simulink model "ROBOT_CONTROL_K2"  (R2023a)
settings: Solver=VariableStepAuto  StartTime=0.0  StopTime=10  RelTol=1e-3
values from neighbouring files (symbols this model uses):
  Bm = 0.015    [ROBOT_CONTROL.m]    (also in collaborative_class_main.m)
  g = 9.81    [ROBOT_CONTROL.m]    (also in collaborative_class_main.m)
  Jl = 4e-4    (= 0.0004)    [ROBOT_CONTROL.m]    (also in collaborative_class_main.m)
  Jm = 4e-4    (= 0.0004)    [ROBOT_CONTROL.m]    (also in collaborative_class_main.m)
  k = 0.8    [ROBOT_CONTROL.m]    (also in collaborative_class_main.m)
  l = 0.3    [ROBOT_CONTROL.m]    (also in collaborative_class_main.m)
  m = 0.3    [ROBOT_CONTROL.m]    (also in collaborative_class_main.m)
  u_bar = m*g*l*cos(x2_bar)    [ROBOT_CONTROL.m]
undefined symbols (not defined in the file or in its folder): const, Kv_tilde
settings Model: Creator=Kevin  LastModifiedBy=alexz

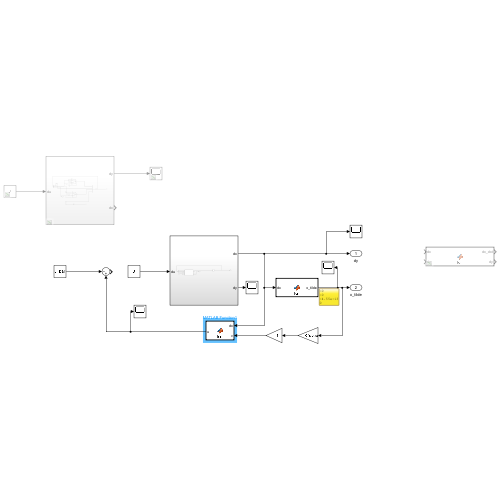
[thumbnail: Simulink's stored preview of the top-level diagram]
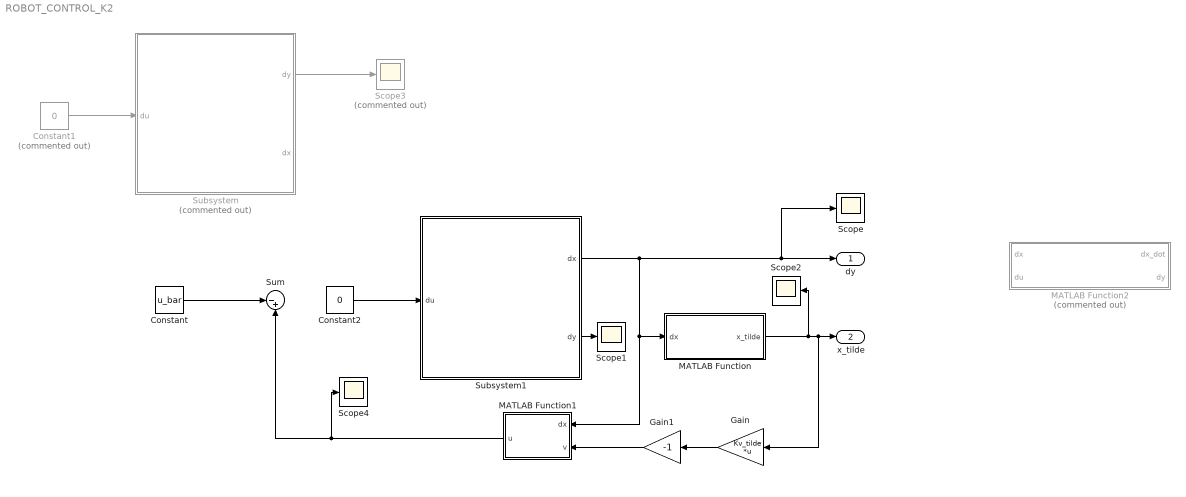
== system ROBOT_CONTROL_K2 ==
  Constant : Constant  Value=u_bar
  Constant1 : Constant  Commented=on  Value=0
  Constant2 : Constant  Value=0
  Gain : Gain  Gain=Kv_tilde  Multiplication=Matrix(K*u) (u vector)
  Gain1 : Gain  Gain=-1
  MATLAB Function : MATLAB Function  TreatAsAtomicUnit=on
  MATLAB Function1 : MATLAB Function  TreatAsAtomicUnit=on
  MATLAB Function2 : MATLAB Function  Commented=on  TreatAsAtomicUnit=on
  Scope{,1..2,4} (4 alike) : Scope
  Scope3 : Scope  Commented=on
  Subsystem : Subsystem  Commented=on
  Subsystem1 : Subsystem
  Sum : Sum  Inputs=|-+
  dy : Outport
  x_tilde : Outport  Port=2
  wires:
  Subsystem1/1(dx) -> MATLAB Function1/1(dx), MATLAB Function/1(dx), Scope/1, dy/1
  MATLAB Function/1(x_tilde) -> Scope2/1, Gain/1, x_tilde/1
  Gain/1 -> Gain1/1
  MATLAB Function1/1(u) -> Scope4/1, Sum/2
  Constant/1 -> Sum/1
  Gain1/1 -> MATLAB Function1/2(v)
  Subsystem1/2(dy) -> Scope1/1
  Constant1/1 -> Subsystem/1(du)
  Subsystem/1(dy) -> Scope3/1
  Constant2/1 -> Subsystem1/1(du)

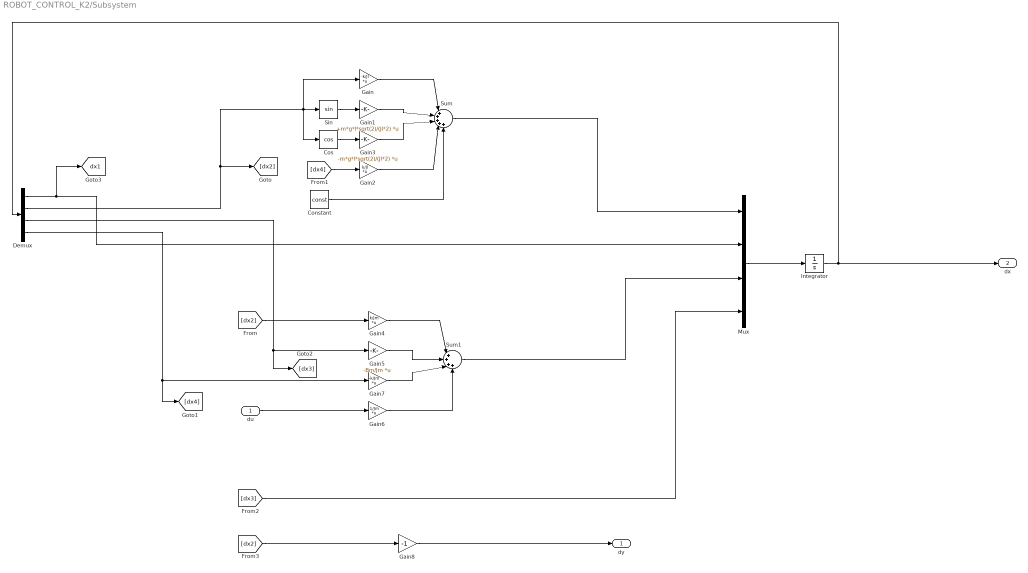
== system ROBOT_CONTROL_K2/Subsystem ==
  du : Inport
  Constant : Constant  Value=const
  Cos : Trigonometry  Operator=cos
  Demux : Demux
  Gain : Gain  Gain=-k/Jl  Multiplication=Matrix(K*u) (u vector)
  Gain1 : Gain  Gain=+m*g*l*sqrt(2)/(Jl*2)  Multiplication=Matrix(K*u) (u vector)
  Gain2 : Gain  Gain=k/Jl  Multiplication=Matrix(K*u) (u vector)
  Gain3 : Gain  Gain=-m*g*l*sqrt(2)/(Jl*2)  Multiplication=Matrix(K*u) (u vector)
  Gain4 : Gain  Gain=k/Jm  Multiplication=Matrix(K*u) (u vector)
  Gain5 : Gain  Gain=-Bm/Jm  Multiplication=Matrix(K*u) (u vector)
  Gain6 : Gain  Gain=1/Jm  Multiplication=Matrix(K*u) (u vector)
  Gain7 : Gain  Gain=-k/Jm  Multiplication=Matrix(K*u) (u vector)
  Gain8 : Gain  Gain=-1
  Integrator : Integrator
  Mux : Mux
  Sin : Trigonometry
  Sum : Sum  Inputs=|+++++
  Sum1 : Sum  Inputs=|++++
  dy : Outport
  dx : Outport  Port=2
  tag scope: dx1=global
  wires:
  [dx2] -> Gain4/1
  Gain6/1 -> Sum1/4
  Gain8/1 -> dy/1
  Demux/2 -> [dx2], Gain/1, Sin/1, Cos/1
  Gain1/1 -> Sum/2
  Constant/1 -> Sum/5
  Cos/1 -> Gain3/1
  Demux/3 -> [dx3], Gain5/1
  [dx4] -> Gain2/1
  Gain7/1 -> Sum1/3
  Sin/1 -> Gain1/1
  Demux/4 -> Gain7/1, [dx4]
  Gain3/1 -> Sum/3
  Sum1/1 -> Mux/3
  Gain4/1 -> Sum1/1
  Gain/1 -> Sum/1
  Gain5/1 -> Sum1/2
  Sum/1 -> Mux/1
  Gain2/1 -> Sum/4
  [dx3] -> Mux/4
  du/1 -> Gain6/1
  [dx2] -> Gain8/1
  Mux/1 -> Integrator/1
  Demux/1 -> [dx1], Mux/2
  Integrator/1 -> dx/1, Demux/1

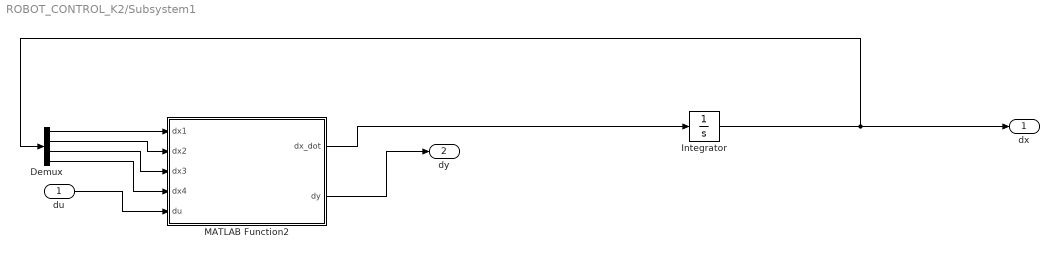
== system ROBOT_CONTROL_K2/Subsystem1 ==
  du : Inport
  Demux : Demux
  Integrator : Integrator
  MATLAB Function2 : MATLAB Function  TreatAsAtomicUnit=on
  dx : Outport
  dy : Outport  Port=2
  wires:
  Integrator/1 -> Demux/1, dx/1
  du/1 -> MATLAB Function2/5(du)
  MATLAB Function2/2(dy) -> dy/1
  MATLAB Function2/1(dx_dot) -> Integrator/1
  Demux/1 -> MATLAB Function2/1(dx1)
  Demux/2 -> MATLAB Function2/2(dx2)
  Demux/3 -> MATLAB Function2/3(dx3)
  Demux/4 -> MATLAB Function2/4(dx4)

== matlab function ROBOT_CONTROL_K2/MATLAB Function ==
  data: dx input; x_tilde output
function x_tilde  = fcn(dx)

dx1 = dx(1);
dx2 = dx(2);
dx3 = dx(3);
dx4 = dx(4);
k = 0.8;
Jm = 4e-4;
Jl= 4e-4;
Bm = 0.015;
Bl = 0;
m = 0.3;
l = 0.3;
g = 9.81;

x1_tilde = -dx2;
x2_tilde = -dx1;
x3_tilde = (k*(pi/4 + dx2))/Jl - (k*(dx4 + sqrt(2)/2*m*g*l/k+pi/4))/Jl + (g*l*m*cos(pi/4 + dx2))/Jl;
x4_tilde = (k*dx1)/Jl - (k*dx3)/Jl - (g*l*m*sin(pi/4 + dx2)*dx1)/Jl;

x_tilde = zeros(length(dx),1);
x_tilde(1) = x1_tilde;
x_tilde(2) = x2_tilde;
x_tilde(3) = x3_tilde;
x_tilde(4) = x4_tilde;

== matlab function ROBOT_CONTROL_K2/MATLAB Function1 ==
  data: dx input; u output; v input
function u  = fcn(dx, v)

%v = 0;
k = 0.8;
Jm = 4e-4;
Jl= 4e-4;
Bm = 0.015;
m = 0.3;
l = 0.3;
g = 9.81;

x1_bar = 0;
x2_bar = pi/4;
x3_bar = 0;
x4_bar = m*g*l*cos(x2_bar)/k + x2_bar;

x1 = dx(1)+x1_bar;
x2 = dx(1)+x2_bar;
x3 = dx(1)+x3_bar;
x4 = dx(1)+x4_bar;

u = ((Jl*Jm)/k)*(-v+(g*l*m*sin(x2*(k*x2 - k*x4 + g*l*m*cos(x2)))/Jl^2 - (- Bm*x3 + k*x2 - k*x4))/(Jl*Jm) - (k*(k*x2 - k*x4 + g*l*m*cos(x2)))/Jl^2 - (g*l*m*cos(x2)*x1^2)/Jl);

== matlab function ROBOT_CONTROL_K2/MATLAB Function2 ==
  data: dx input; du input; dx_dot output; dy output
function [dx_dot, dy]  = fcn(dx, du)

k = 0.8;
Jm = 4e-4;
Jl= 4e-4;
Bm = 0.015;
Bl = 0;
m = 0.3;
l = 0.3;
g = 9.81;
x1_bar = 0;
x2_bar = pi/4;
x3_bar = 0;
x4_bar = m*g*l*cos(x2_bar)/k + x2_bar;
u_bar= m*g*l*cos(x2_bar);

dx1 = dx(1);
dx2 = dx(2);
dx3 = dx(3);
dx4 = dx(4);

dx1_dot = -k/Jl*(dx2+x2_bar)-m*g*l/Jl*(cos(dx2+x2_bar))+k/Jl*(dx4+x4_bar);
dx2_dot = dx1+x1_bar;
dx3_dot = k/Jm*(dx2+x2_dot)-Bm/Jm*(dx3+x3_bar)-k/Jm*(dx4+x4_bar)+1/Jm*(du+u_bar);
dx4_dot = dx3+x3_bar;
dy = pi/4 - (dx2+x2_bar);

dx_dot = zeros(4,1);
dx_dot(1) = dx1_dot;
dx_dot(2) = dx2_dot;
dx_dot(3) = dx3_dot;
dx_dot(4) = dx4_dot;

== matlab function ROBOT_CONTROL_K2/Subsystem1/MATLAB Function2 ==
  data: dx1 input; dx2 input; dx3 input; dx4 input; du input; dx_dot output; dy output
function [dx_dot, dy]  = fcn(dx1,dx2,dx3,dx4, du)

k = 0.8;
Jm = 4e-4;
Jl= 4e-4;
Bm = 0.015;
Bl = 0;
m = 0.3;
l = 0.3;
g = 9.81;
x1_bar = 0;
x2_bar = pi/4;
x3_bar = 0;
x4_bar = m*g*l*cos(x2_bar)/k + x2_bar;
u_bar= m*g*l*cos(x2_bar);


dx1_dot = -k/Jl*(dx2+x2_bar)-m*g*l/Jl*(cos(dx2+x2_bar))+k/Jl*(dx4+x4_bar);
dx2_dot = dx1+x1_bar;
dx3_dot = k/Jm*(dx2+x2_bar)-Bm/Jm*(dx3+x3_bar)-k/Jm*(dx4+x4_bar)+1/Jm*(du+u_bar);
dx4_dot = dx3+x3_bar;
dy = pi/4 - (dx2+x2_bar);

dx_dot = zeros(1,4);
dx_dot(1) = dx1_dot;
dx_dot(2) = dx2_dot;
dx_dot(3) = dx3_dot;
dx_dot(4) = dx4_dot;
